simulink model "hall_filter_demo_noreset"  (R2024b)
settings: Solver=VariableStepAuto  StartTime=0.0  StopTime=0.5  RelTol=1e-3
undefined symbols (not defined in the file or in its folder): DiscIntNeverNeededParam, period
libraries: simulink x1, embmathops x1
settings Model: PacingRate=0.500000  Creator=baolo  LastModifiedBy=baolo
settings SolverCC: AutoInsertRateTranBlk=on

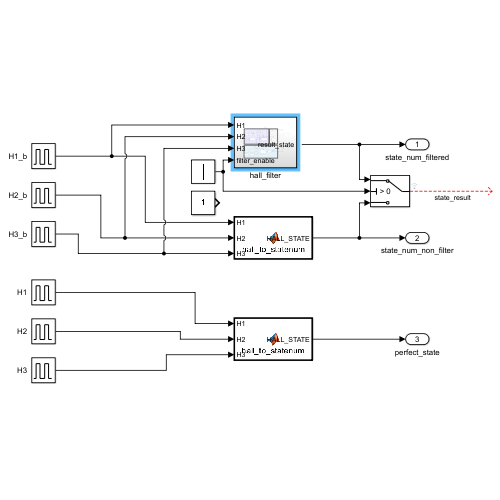
[thumbnail: Simulink's stored preview of the top-level diagram]
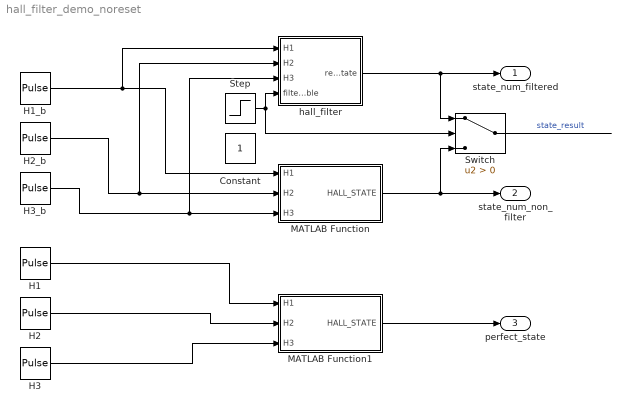
== system hall_filter_demo_noreset ==
  Constant : Constant
  H1 : DiscretePulseGenerator  PulseType=Time based  Period=period  PulseWidth=50
  H1_b : DiscretePulseGenerator  PulseType=Time based  Period=period  PulseWidth=50  PhaseDelay=period*(2/360)
  H2 : DiscretePulseGenerator  PulseType=Time based  Period=period  PulseWidth=50  PhaseDelay=period*1/3
  H2_b : DiscretePulseGenerator  PulseType=Time based  Period=period  PulseWidth=50  PhaseDelay=period*(1/3 + 4/360)
  H3 : DiscretePulseGenerator  PulseType=Time based  Period=period  PulseWidth=50  PhaseDelay=period*2/3
  H3_b : DiscretePulseGenerator  PulseType=Time based  Period=period  PulseWidth=50  PhaseDelay=period*(2/3+6/360)
  MATLAB Function : MATLAB Function  TreatAsAtomicUnit=on
  MATLAB Function1 : MATLAB Function  TreatAsAtomicUnit=on
  Step : Step  Time=0.2  SampleTime=0
  Switch : Switch  Criteria=u2 > Threshold  SaturateOnIntegerOverflow=off  InputSameDT=off
  hall_filter : Subsystem
  state_num_filtered : Outport
  state_num_non_filter : Outport  Port=2
  perfect_state : Outport  Port=3
  wires:
  MATLAB Function/1(HALL_STATE) -> Switch/3, state_num_non_filter/1
  hall_filter/1(result_state) -> Switch/1, state_num_filtered/1
  H1/1 -> MATLAB Function1/1(H1)
  H2/1 -> MATLAB Function1/2(H2)
  H3/1 -> MATLAB Function1/3(H3)
  MATLAB Function1/1(HALL_STATE) -> perfect_state/1
  H1_b/1 -> hall_filter/1(H1), MATLAB Function/1(H1)
  H2_b/1 -> hall_filter/2(H2), MATLAB Function/2(H2)
  H3_b/1 -> hall_filter/3(H3), MATLAB Function/3(H3)
  Step/1 -> Switch/2, hall_filter/4(filter_enable)
  Switch/1 -> ?  "state_result"

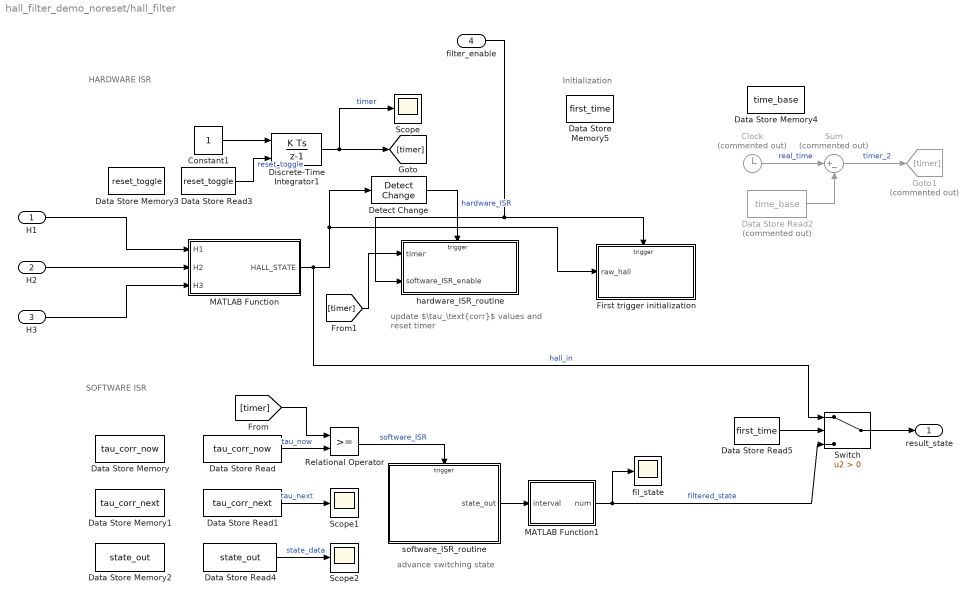
== system hall_filter_demo_noreset/hall_filter ==
  note: Initialization
  note: SOFTWARE ISR
  note: HARDWARE ISR
  note: update $\tau_\text{corr}$ values and reset timer
  note: advance switching state
  H1 : Inport
  H2 : Inport  Port=2
  H3 : Inport  Port=3
  filter_enable : Inport  Port=4
  Clock : Clock  Commented=on
  Constant1 : Constant
  Data Store Memory : DataStoreMemory  DataStoreName=tau_corr_now  WriteAfterWriteMsg=warning  InitialValue=-1  ShowAdditionalParam=off
  Data Store Memory1 : DataStoreMemory  DataStoreName=tau_corr_next  WriteAfterWriteMsg=warning  InitialValue=-1  ShowAdditionalParam=off
  Data Store Memory2 : DataStoreMemory  DataStoreName=state_out  WriteAfterWriteMsg=warning  InitialValue=2  ShowAdditionalParam=off
  Data Store Memory3 : DataStoreMemory  DataStoreName=reset_toggle  WriteAfterWriteMsg=warning  ShowAdditionalParam=off
  Data Store Memory4 : DataStoreMemory  DataStoreName=time_base  WriteAfterWriteMsg=warning  ShowAdditionalParam=off
  Data Store Memory5 : DataStoreMemory  DataStoreName=first_time  WriteAfterWriteMsg=warning  InitialValue=1  ShowAdditionalParam=off
  Data Store Read : DataStoreRead  DataStoreName=tau_corr_now  IndexOptions=Index vector (dialog)  Indices=1  OutputSizes=1
  Data Store Read1 : DataStoreRead  DataStoreName=tau_corr_next  IndexOptions=Index vector (dialog)  Indices=1  OutputSizes=1
  Data Store Read2 : DataStoreRead  Commented=on  DataStoreName=time_base  IndexOptions=Index vector (dialog)  Indices=1  OutputSizes=1
  Data Store Read3 : DataStoreRead  DataStoreName=reset_toggle  IndexOptions=Index vector (dialog)  Indices=1  OutputSizes=1
  Data Store Read4 : DataStoreRead  DataStoreName=state_out  IndexOptions=Index vector (dialog)  Indices=1  OutputSizes=1
  Data Store Read5 : DataStoreRead  DataStoreName=first_time  IndexOptions=Index vector (dialog)  Indices=1  OutputSizes=1
  Detect Change : simulink/Logic and Bit Operations/Detect Change  vinit=0  OutDataTypeStr=boolean
  Discrete-Time Integrator1 : DiscreteIntegrator  ExternalReset=either  SampleTime=1/(1e6)  ICPrevOutput=DiscIntNeverNeededParam  ICPrevScaledInput=DiscIntNeverNeededParam
  First trigger initialization : Subsystem  TreatAsAtomicUnit=on
  Goto1 : Goto  Commented=on  GotoTag=timer
  MATLAB Function : MATLAB Function  TreatAsAtomicUnit=on
  MATLAB Function1 : MATLAB Function  TreatAsAtomicUnit=on
  Relational Operator : RelationalOperator  OutDataTypeStr=boolean  RndMeth=Simplest  InputSameDT=off
  Scope : Scope
  Scope1 : Scope
  Scope2 : Scope
  Sum : Sum  Commented=on  Inputs=|+-
  Switch : Switch  Criteria=u2 > Threshold  SaturateOnIntegerOverflow=off  InputSameDT=off
  fil_state : Scope
  hardware_ISR_routine : Subsystem  Priority=1
  software_ISR_routine : Subsystem  Priority=10  TreatAsAtomicUnit=on
  result_state : Outport
  wires:
  Discrete-Time Integrator1/1 -> [timer], Scope/1  "timer"
  Relational Operator/1 -> software_ISR_routine/Trigger  "software_ISR"
  Constant1/1 -> Discrete-Time Integrator1/1
  [timer] -> Relational Operator/1
  software_ISR_routine/1(state_out) -> MATLAB Function1/1(interval)
  MATLAB Function/1(HALL_STATE) -> Switch/1, Detect Change/1, First trigger initialization/1(raw_hall)  "hall_in"
  Data Store Read3/1 -> Discrete-Time Integrator1/2  "reset_toggle"
  Data Store Read1/1 -> Scope1/1  "tau_next"
  Data Store Read/1 -> Relational Operator/2  "tau_now"
  H3/1 -> MATLAB Function/3(H3)
  H2/1 -> MATLAB Function/2(H2)
  H1/1 -> MATLAB Function/1(H1)
  MATLAB Function1/1(num) -> fil_state/1, Switch/3  "filtered_state"
  Detect Change/1 -> hardware_ISR_routine/Trigger  "hardware_ISR"
  Data Store Read4/1 -> Scope2/1  "state_data"
  filter_enable/1 -> First trigger initialization/Trigger, hardware_ISR_routine/2(software_ISR_enable)
  Clock/1 -> Sum/1  "real_time"
  [timer] -> hardware_ISR_routine/1(timer)
  Data Store Read2/1 -> Sum/2
  Sum/1 -> Goto1/1  "timer_2"
  Data Store Read5/1 -> Switch/2
  Switch/1 -> result_state/1

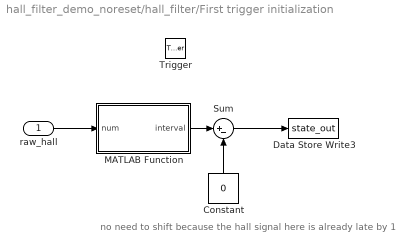
== system hall_filter_demo_noreset/hall_filter/First trigger initialization ==
  note: no need to shift because the hall signal here is already late by 1
  raw_hall : Inport
  Trigger : TriggerPort  VariantControl=(inherit)  PortDimensions=1
  Constant : Constant  Value=0
  Data Store Write3 : DataStoreWrite  DataStoreName=state_out  IndexOptions=Index vector (dialog)  Indices=1  OutputSizes=1
  MATLAB Function : MATLAB Function  TreatAsAtomicUnit=on
  Sum : Sum  Inputs=|+-
  wires:
  raw_hall/1 -> MATLAB Function/1(num)
  MATLAB Function/1(interval) -> Sum/1
  Sum/1 -> Data Store Write3/1
  Constant/1 -> Sum/2

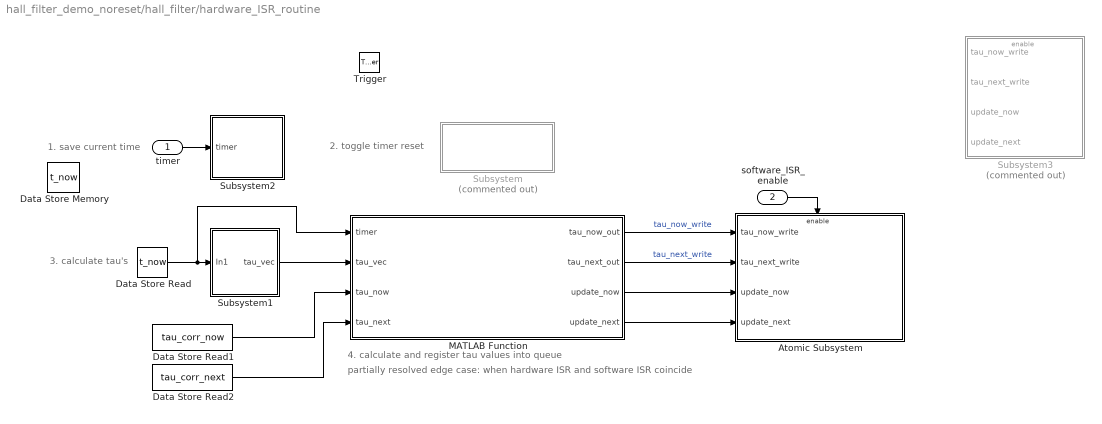
== system hall_filter_demo_noreset/hall_filter/hardware_ISR_routine ==
  note: partially resolved edge case: when hardware ISR and software ISR coincide
  note: 2. toggle timer reset
  note: 3. calculate tau's
  note: 4. calculate and register tau values into queue
  note: 1. save current time
  timer : Inport
  software_ISR_enable : Inport  Port=2
  Trigger : TriggerPort  VariantControl=(inherit)  PortDimensions=1
  Atomic Subsystem : Subsystem  Priority=5  TreatAsAtomicUnit=on
  Data Store Memory : DataStoreMemory  DataStoreName=t_now  WriteAfterWriteMsg=warning  ShowAdditionalParam=off
  Data Store Read : DataStoreRead  DataStoreName=t_now  IndexOptions=Index vector (dialog)  Indices=1  OutputSizes=1
  Data Store Read1 : DataStoreRead  DataStoreName=tau_corr_now  IndexOptions=Index vector (dialog)  Indices=1  OutputSizes=1
  Data Store Read2 : DataStoreRead  DataStoreName=tau_corr_next  IndexOptions=Index vector (dialog)  Indices=1  OutputSizes=1
  MATLAB Function : MATLAB Function  Priority=4  TreatAsAtomicUnit=on
  Subsystem : Subsystem  Priority=2  Commented=on
  Subsystem1 : Subsystem  Priority=3
  Subsystem2 : Subsystem  Priority=1
  Subsystem3 : Subsystem  Priority=5  Commented=on
  wires:
  Data Store Read/1 -> MATLAB Function/1(timer), Subsystem1/1(In1)
  Data Store Read1/1 -> MATLAB Function/3(tau_now)
  Data Store Read2/1 -> MATLAB Function/4(tau_next)
  timer/1 -> Subsystem2/1(timer)
  Subsystem1/1(tau_vec) -> MATLAB Function/2(tau_vec)
  MATLAB Function/1(tau_now_out) -> Atomic Subsystem/1(tau_now_write)  "tau_now_write"
  MATLAB Function/2(tau_next_out) -> Atomic Subsystem/2(tau_next_write)  "tau_next_write"
  software_ISR_enable/1 -> Atomic Subsystem/Enable
  MATLAB Function/3(update_now) -> Atomic Subsystem/3(update_now)
  MATLAB Function/4(update_next) -> Atomic Subsystem/4(update_next)

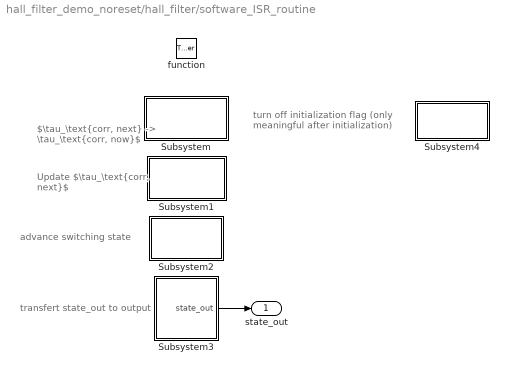
== system hall_filter_demo_noreset/hall_filter/software_ISR_routine ==
  note: turn off initialization flag
      | (only meaningful after initialization)
  note: advance switching state
  note: $\tau_\text{corr, next} -> \tau_\text{corr, now}$
  note: Update $\tau_\text{corr, next}$
  note: transfert state_out to output
  function : TriggerPort  VariantControl=(inherit)
  Subsystem : Subsystem  Priority=11
  Subsystem1 : Subsystem  Priority=12
  Subsystem2 : Subsystem  Priority=13
  Subsystem3 : Subsystem  Priority=14
  Subsystem4 : Subsystem  Priority=11
  state_out : Outport
  wires:
  Subsystem3/1(state_out) -> state_out/1

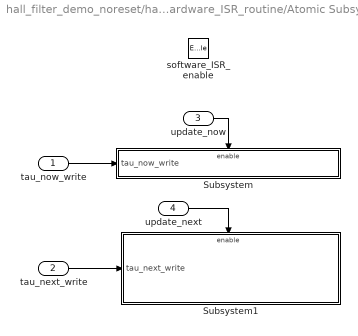
== system hall_filter_demo_noreset/hall_filter/hardware_ISR_routine/Atomic Subsystem ==
  tau_now_write : Inport
  tau_next_write : Inport  Port=2
  update_now : Inport  Port=3
  update_next : Inport  Port=4
  software_ISR_enable : EnablePort
  Subsystem : Subsystem
  Subsystem1 : Subsystem
  wires:
  tau_next_write/1 -> Subsystem1/1(tau_next_write)
  update_now/1 -> Subsystem/Enable
  update_next/1 -> Subsystem1/Enable
  tau_now_write/1 -> Subsystem/1(tau_now_write)

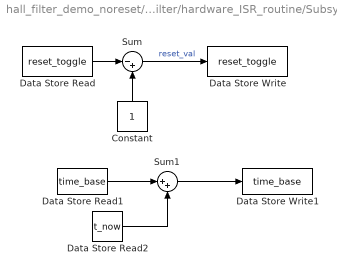
== system hall_filter_demo_noreset/hall_filter/hardware_ISR_routine/Subsystem ==
  Constant : Constant
  Data Store Read : DataStoreRead  DataStoreName=reset_toggle  IndexOptions=Index vector (dialog)  Indices=1  OutputSizes=1
  Data Store Read1 : DataStoreRead  DataStoreName=time_base  IndexOptions=Index vector (dialog)  Indices=1  OutputSizes=1
  Data Store Read2 : DataStoreRead  DataStoreName=t_now  IndexOptions=Index vector (dialog)  Indices=1  OutputSizes=1
  Data Store Write : DataStoreWrite  DataStoreName=reset_toggle  IndexOptions=Index vector (dialog)  Indices=1  OutputSizes=1
  Data Store Write1 : DataStoreWrite  DataStoreName=time_base  IndexOptions=Index vector (dialog)  Indices=1  OutputSizes=1
  Sum : Sum  Inputs=|-+
  Sum1 : Sum  Inputs=|++
  wires:
  Sum/1 -> Data Store Write/1  "reset_val"
  Data Store Read/1 -> Sum/1
  Constant/1 -> Sum/2
  Data Store Read1/1 -> Sum1/1
  Sum1/1 -> Data Store Write1/1
  Data Store Read2/1 -> Sum1/2

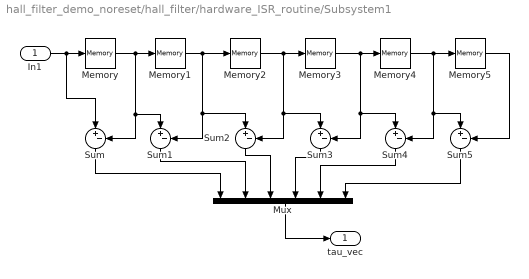
== system hall_filter_demo_noreset/hall_filter/hardware_ISR_routine/Subsystem1 ==
  In1 : Inport
  Memory{,1..5} (6 alike) : Memory  InheritSampleTime=on
  Mux : Mux  Inputs=6
  Sum{,1..5} (6 alike) : Sum  Inputs=|+-
  tau_vec : Outport
  wires:
  Memory1/1 -> Sum1/2, Sum2/1, Memory2/1
  Memory/1 -> Sum1/1, Sum/2, Memory1/1
  Memory2/1 -> Sum3/1, Sum2/2, Memory3/1
  In1/1 -> Sum/1, Memory/1
  Memory3/1 -> Sum4/1, Sum3/2, Memory4/1
  Memory4/1 -> Memory5/1, Sum5/1, Sum4/2
  Mux/1 -> tau_vec/1
  Memory5/1 -> Sum5/2
  Sum/1 -> Mux/1
  Sum1/1 -> Mux/2
  Sum2/1 -> Mux/3
  Sum3/1 -> Mux/4
  Sum4/1 -> Mux/5
  Sum5/1 -> Mux/6

== system hall_filter_demo_noreset/hall_filter/hardware_ISR_routine/Subsystem2 ==
  timer : Inport
  Data Store Write2 : DataStoreWrite  DataStoreName=t_now  IndexOptions=Index vector (dialog)  Indices=1  OutputSizes=1
  wires:
  timer/1 -> Data Store Write2/1

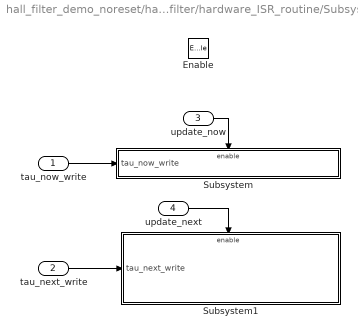
== system hall_filter_demo_noreset/hall_filter/hardware_ISR_routine/Subsystem3 ==
  tau_now_write : Inport
  tau_next_write : Inport  Port=2
  update_now : Inport  Port=3
  update_next : Inport  Port=4
  Enable : EnablePort
  Subsystem : Subsystem
  Subsystem1 : Subsystem
  wires:
  tau_now_write/1 -> Subsystem/1(tau_now_write)
  tau_next_write/1 -> Subsystem1/1(tau_next_write)
  update_now/1 -> Subsystem/Enable
  update_next/1 -> Subsystem1/Enable

== system hall_filter_demo_noreset/hall_filter/software_ISR_routine/Subsystem ==
  Data Store Read : DataStoreRead  DataStoreName=tau_corr_next  IndexOptions=Index vector (dialog)  Indices=1  OutputSizes=1
  Data Store Write : DataStoreWrite  DataStoreName=tau_corr_now  IndexOptions=Index vector (dialog)  Indices=1  OutputSizes=1
  wires:
  Data Store Read/1 -> Data Store Write/1

== system hall_filter_demo_noreset/hall_filter/software_ISR_routine/Subsystem1 ==
  Constant : Constant  Value=-1
  Data Store Write1 : DataStoreWrite  DataStoreName=tau_corr_next  IndexOptions=Index vector (dialog)  Indices=1  OutputSizes=1
  wires:
  Constant/1 -> Data Store Write1/1

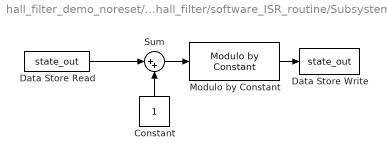
== system hall_filter_demo_noreset/hall_filter/software_ISR_routine/Subsystem2 ==
  Constant : Constant
  Data Store Read : DataStoreRead  DataStoreName=state_out  IndexOptions=Index vector (dialog)  Indices=1  OutputSizes=1
  Data Store Write : DataStoreWrite  DataStoreName=state_out  IndexOptions=Index vector (dialog)  Indices=1  OutputSizes=1
  Modulo by Constant : embmathops/Modulo by Constant  Denominator=6  SimulateUsing=Code generation
      settings: LibrarySourceBlock=embeddedMathLib/Modulo by Constant
  Sum : Sum  Inputs=|++
  wires:
  Constant/1 -> Sum/2
  Data Store Read/1 -> Sum/1
  Sum/1 -> Modulo by Constant/1
  Modulo by Constant/1 -> Data Store Write/1

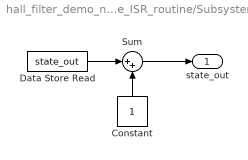
== system hall_filter_demo_noreset/hall_filter/software_ISR_routine/Subsystem3 ==
  Constant : Constant
  Data Store Read : DataStoreRead  DataStoreName=state_out  IndexOptions=Index vector (dialog)  Indices=1  OutputSizes=1
  Sum : Sum  Inputs=|++
  state_out : Outport
  wires:
  Data Store Read/1 -> Sum/1
  Sum/1 -> state_out/1
  Constant/1 -> Sum/2

== system hall_filter_demo_noreset/hall_filter/software_ISR_routine/Subsystem4 ==
  Constant : Constant  Value=0
  Data Store Write : DataStoreWrite  DataStoreName=first_time  IndexOptions=Index vector (dialog)  Indices=1  OutputSizes=1
  wires:
  Constant/1 -> Data Store Write/1

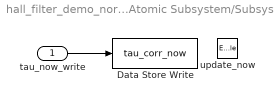
== system hall_filter_demo_noreset/hall_filter/hardware_ISR_routine/Atomic Subsystem/Subsystem ==
  tau_now_write : Inport
  update_now : EnablePort
  Data Store Write : DataStoreWrite  DataStoreName=tau_corr_now  IndexOptions=Index vector (dialog)  Indices=1  OutputSizes=1
  wires:
  tau_now_write/1 -> Data Store Write/1

== system hall_filter_demo_noreset/hall_filter/hardware_ISR_routine/Atomic Subsystem/Subsystem1 ==
  tau_next_write : Inport
  update_next : EnablePort
  Data Store Write1 : DataStoreWrite  DataStoreName=tau_corr_next  IndexOptions=Index vector (dialog)  Indices=1  OutputSizes=1
  wires:
  tau_next_write/1 -> Data Store Write1/1

== system hall_filter_demo_noreset/hall_filter/hardware_ISR_routine/Subsystem3/Subsystem ==
  tau_now_write : Inport
  update_now : EnablePort
  Data Store Write : DataStoreWrite  DataStoreName=tau_corr_now  IndexOptions=Index vector (dialog)  Indices=1  OutputSizes=1
  wires:
  tau_now_write/1 -> Data Store Write/1

== system hall_filter_demo_noreset/hall_filter/hardware_ISR_routine/Subsystem3/Subsystem1 ==
  tau_next_write : Inport
  update_next : EnablePort
  Data Store Write1 : DataStoreWrite  DataStoreName=tau_corr_next  IndexOptions=Index vector (dialog)  Indices=1  OutputSizes=1
  wires:
  tau_next_write/1 -> Data Store Write1/1

== matlab function hall_filter_demo_noreset/hall_filter/hardware_ISR_routine/MATLAB Function ==
  data: timer input; tau_now_out output; tau_vec input; tau_now input; tau_next input; tau_next_out output; update_now output; update_next output
function [tau_now_out, tau_next_out, update_now, update_next] = update_tau_vals_conditional_sim(timer, tau_vec, tau_now, tau_next)
[tau_now_out, tau_next_out, update_now, update_next] = update_tau_vals_conditional(timer, tau_vec, tau_now, tau_next);

== matlab function hall_filter_demo_noreset/hall_filter/MATLAB Function ==
  data: H1 input; HALL_STATE output; H2 input; H3 input
function HALL_STATE = hall_to_statenum(H1,H2,H3)
HALL_STATE = 4*H1 + 2*H2 + H3;

== matlab function hall_filter_demo_noreset/MATLAB Function ==
  data: H1 input; HALL_STATE output; H2 input; H3 input
function HALL_STATE = hall_to_statenum(H1,H2,H3)
HALL_STATE = 4*H1 + 2*H2 + H3;

== matlab function hall_filter_demo_noreset/MATLAB Function1 ==
  data: H1 input; HALL_STATE output; H2 input; H3 input
function HALL_STATE = hall_to_statenum(H1,H2,H3)
HALL_STATE = 4*H1 + 2*H2 + H3;

== matlab function hall_filter_demo_noreset/hall_filter/MATLAB Function1 ==
  data: interval input; num output
function num = interval_to_num(interval)
DICT = [4,6,2,3,1,5];
if interval == 0
    num = 0;
else
    num = DICT(interval);
end

== matlab function hall_filter_demo_noreset/hall_filter/First trigger initialization/MATLAB Function ==
  data: num input; interval output
function interval = num_to_interval(num)
DICT = [5,3,4,1,6,2];
interval = DICT(num);
